simulink model "Master2021b"  (R2021b)
settings: Solver=ode23t  StartTime=0.0  StopTime=simtime  MaxStep=1  RelTol=1e-3
values from neighbouring files (symbols this model uses):
  Af = 1.8    [Akik_DriveCycle_Model_price.m]
  B = 0.0001    [Akik_DriveCycle_Model_price.m]
  Cd = 0.3    [Akik_DriveCycle_Model_price.m]
  Conv_eff = 0.9    [Akik_DriveCycle_Model_price.m]
  fr = 0.015    [Akik_DriveCycle_Model_price.m]
  g = 9.81    [Akik_DriveCycle_Model_price.m]
  Gain = 1    [Akik_DriveCycle_Model_price.m]
  Gr = 9.7    [Akik_DriveCycle_Model_price.m]
  Initial_SOC = 1    [Akik_DriveCycle_Model_price.m]
  J = 1.7    [Akik_DriveCycle_Model_price.m]
  Kd = 0    [Akik_DriveCycle_Model_price.m]
  Ke = 0.33    [Akik_DriveCycle_Model_price.m]
  Ki = 0.05    [Akik_DriveCycle_Model_price.m]
  Kp = 0.3    [Akik_DriveCycle_Model_price.m]
  Kt = 0.33    [Akik_DriveCycle_Model_price.m]
  L = 9e-5    (= 9e-05)    [Akik_DriveCycle_Model_price.m]
  max_brakeT = 3000    [Akik_DriveCycle_Model_price.m]
  Mv = 1500    [Akik_DriveCycle_Model_price.m]
  Qmax = 150    [Akik_DriveCycle_Model_price.m]
  r = 0.35    [Akik_DriveCycle_Model_price.m]
  Ra = 0.55    [Akik_DriveCycle_Model_price.m]
  Rho = 1.2    [Akik_DriveCycle_Model_price.m]
undefined symbols (not defined in the file or in its folder): Ion, Lithium
libraries: simulink x3, spsBatteryLib x1, spsControlledCurrentSourceLib x1, spsStairGeneratorLib x1, spspowerguiLib x1
settings Model: Creator=bkudachi  LastModifiedBy=CP Gaming1
settings DebuggingCC: UnconnectedInputMsg=none  UnconnectedOutputMsg=none  UnconnectedLineMsg=none
settings RTWCC: DLArmComputeVersion=20.02.1

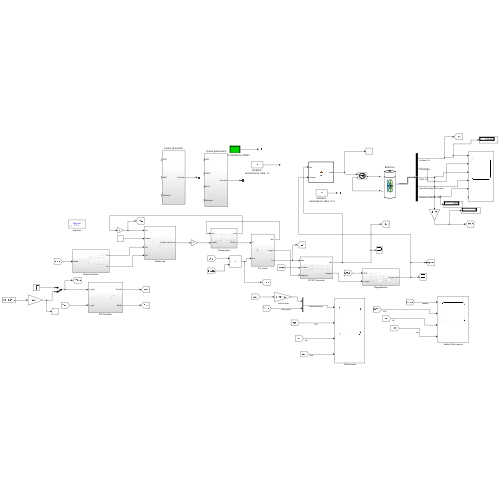
[thumbnail: Simulink's stored preview of the top-level diagram]
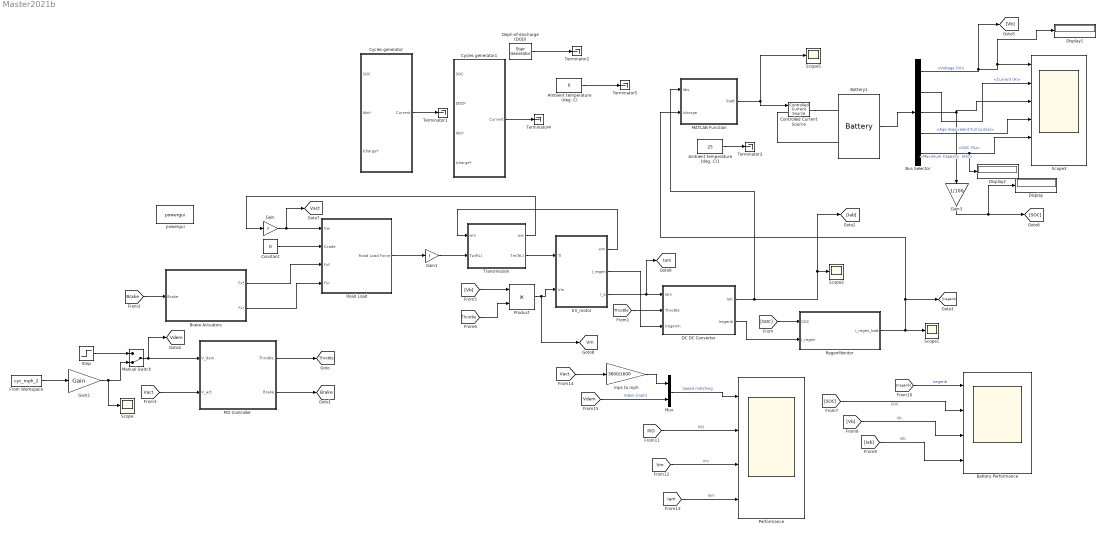
== system Master2021b ==
  " Performance" : Scope  NumInputPorts=4
  Ambient temperature (deg. C) : Constant  Value=0
  Ambient temperature (deg. C)1 : Constant  Value=25
  Battery Performance : Scope  NumInputPorts=4
  Battery1 : spsBatteryLib/Battery  BatType=Lithium-Ion  ShowTempParam=off  ThermalPreset=no  ShowAgeParam=on  NomV=380  NomQ=Qmax  SOC=Initial_SOC*100  Batt_Tr=90  PresetModel=on  MaxQ=150  MinV=285  FullV=442.3151  Dis_rate=65.2174  R=0.025333  Normal_OP=135.6522  expZone="[410.5466      7.369565]"  current=[0.15 1.3 3.25]  Units=Ampere-hour  Tci=25  NomT=20  T2=0  MaxQ2=36  FullV2=13  Normal_OP2=11.7  expZone2="[12.67            4]"  Rca=0.6411  ti=4880  Dp=0  Neq0=0  Tsim=30  Ta1=23  Qeol=40*0.9  Reol=0.0126*1.2  Char_age=[20, 26]  Dis_age=[20, 80]  N1=1500  N2=10445  N3=1017  N4=1460  Ta2=45  N5=982
  Brake Actuators : Subsystem
  Bus Selector : BusSelector  OutputSignals="Voltage (V),Current (A),SOC (%),Age (Equivalent Full cycles),Maximum Capacity  (Ah)"
  Constant : Constant  Value=0
  Controlled Current Source : spsControlledCurrentSourceLib/Controlled Current Source  Initialize=on  Source_Type=AC  Amplitude=0  Phase=0  Frequency=0  Measurements=None
  Cycles generator : Subsystem
  Cycles generator1 : Subsystem
  DC DC Converter : Subsystem
  Deph-of-discharge (DOD) : spsStairGeneratorLib/Stair Generator  t=[0 50 100]*14400  e=[20 80 20]  Ts=0
  Display : Display
  Display1 : Display
  Display2 : Display
  EV_motor : Subsystem
  From Workspace : FromWorkspace  VariableName=cyc_mph_2
  Gain : Gain  Gain=r
  Gain1 : Gain  Gain=r
  Gain2 : Gain  Gain=Gain
  Gain3 : Gain  Gain=1/100
  MATLAB Function : MATLAB Function  TreatAsAtomicUnit=on
  Manual Switch : ManualSwitch  CurrentSetting=0
  Mux : Mux  Inputs=2
  PID Controller : Subsystem
  Product : Product
  RegenMonitor : Subsystem
  Road Load : Subsystem
  Scope{,1..2,5} (4 alike) : Scope
  Scope3 : Scope  NumInputPorts=6
  Step : Step  Time=0  After=100  SampleTime=0
  Terminator{1..5} (5 alike) : Terminator
  Transmission : Subsystem
  mps to mph : Gain  Gain=3600/1600
  powergui : spspowerguiLib/powergui  Priority=1  SimulationMode=Discrete  SampleTime=.1  frequency=60  Iterations=50  frequencyindice=0  Pbase=100e6  ErrMax=1e-4  UnitsV=kV  UnitsW=MW  buscounter=0  FunctionMessages=off  echomessages=off  EnableUseOfTLC=off  CurrentSourceSwitches=off  DisableSnubberDevices=off  DisableRonSwitches=off  DisableVfSwitches=off  DisplayEquations=off  AutomaticDiscreteSolvers=off  SolverType=Tustin/Backward Euler (TBE)  Interpol=off  ExternalGateDelay=off  methode=off  Ts=100  x0status=blocks  SPID=on  SwTol=0  HookPort=off  NonlinearTolerance=1e-4  nMaxIteration=100  ContinueOnMaxIteration=off  RestoreLinks=warning  ResistiveCurrentMeasurement=off  Frange=[0:2:500]  Ylog=off  Xlog=on  ShowGrid=off  save=off  variable=ZData  structure=0  ZoomFFT=off  StartTime=0.0  cycles=1  DisplayStyle=1  fundamental=60  FreqAxis=off  MaxFrequency=1000  frequencyindicesteady=1  RmsSteady=1  display=off
  tag scope: Brake=global, Iam=global, Throttle=global, Vact=global, Vdem=global, Vm=global
  wires:
  Constant/1 -> Road Load/2(Grade)
  Gain/1 -> [Vact], Road Load/1(Vw)
  Road Load/1(Road Load Force) -> Gain1/1
  Brake Actuators/1(Fxf) -> Road Load/3(Fxf)
  Brake Actuators/2(Fxr) -> Road Load/4(Fxr)
  Transmission/1(ww) -> Gain/1
  Transmission/2(Tm(RL)) -> EV_motor/1(Tl)
  EV_motor/1(wm) -> Transmission/1(wm)
  EV_motor/3(I_a) -> [Iam], DC DC Converter/1(Iam)
  EV_motor/2(I_regen) -> DC DC Converter/3(Iregenm)
  DC DC Converter/2(Iregenb) -> RegenMonitor/2(I_regen)
  [SOC] -> RegenMonitor/1(SOC)
  PID Controller/1(Throttle) -> [Throttle]
  PID Controller/2(Brake) -> [Brake]
  RegenMonitor/1(I_regen_batt) -> MATLAB Function/2(Icharge), [Iregenb], Scope1/1
  DC DC Converter/1(Iab) -> MATLAB Function/1(Idis), [Iab], Scope2/1
  [Throttle] -> DC DC Converter/2(Throttle)
  [Brake] -> Brake Actuators/1(Brake)
  [Vact] -> PID Controller/2(V_act)
  [Vb] -> Product/1
  Product/1 -> [Vm], EV_motor/2(Vm)
  [Throttle] -> Product/2
  [Iab] -> Battery Performance/4  "Iab"
  [Iregenb] -> Battery Performance/1  "Iregenb"
  [PID] -> " Performance"/2  "PID"
  [Vm] -> " Performance"/3  "Vm"
  [Iam] -> " Performance"/4  "Iam"
  [Vact] -> mps to mph/1
  mps to mph/1 -> Mux/1
  Mux/1 -> " Performance"/1  "Speed matching"
  [Vdem] -> Mux/2  "Vdem (mph)"
  Step/1 -> Manual Switch/1
  Manual Switch/1 -> [Vdem], PID Controller/1(V_dem)
  From Workspace/1 -> Gain2/1
  Gain2/1 -> Scope/1, Manual Switch/2
  Gain1/1 -> Transmission/2(Tw(RL))
  Battery1/1 -> Bus Selector/1
  Bus Selector/1 -> [Vb], Display1/1, Scope3/1  "<Voltage (V)>"
  Gain3/1 -> Display/1, [SOC]
  [Vb] -> Battery Performance/3  "Vb"
  [SOC] -> Battery Performance/2  "SOC"
  Deph-of-discharge (DOD)/1 -> Terminator2/1
  Cycles generator/1(Current) -> Terminator1/1
  Cycles generator1/1(Current) -> Terminator4/1
  Ambient temperature (deg. C)/1 -> Terminator5/1
  MATLAB Function/1(ibatt) -> Scope5/1, Controlled Current Source/1
  Bus Selector/2 -> Scope3/2  "<Current (A)>"
  Bus Selector/3 -> Scope3/3, Gain3/1  "<SOC (%)>"
  Ambient temperature (deg. C)1/1 -> Terminator3/1
  Bus Selector/4 -> Scope3/4  "<Age (Equivalent Full cycles)>"
  Bus Selector/5 -> Display2/1, Scope3/5  "<Maximum Capacity  (Ah)>"
  connections:
  Controlled Current Source/RConn1 -- Battery1/LConn2
  Controlled Current Source/LConn1 -- Battery1/LConn1

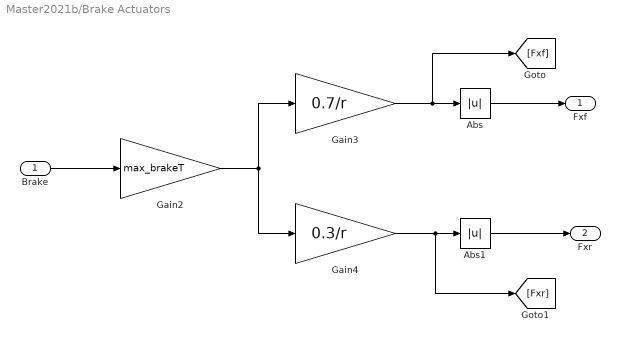
== system Master2021b/Brake Actuators ==
  Brake : Inport
  Abs : Abs
  Abs1 : Abs
  Gain2 : Gain  Gain=max_brakeT
  Gain3 : Gain  Gain=0.7/r
  Gain4 : Gain  Gain=0.3/r
  Fxf : Outport
  Fxr : Outport  Port=2
  wires:
  Gain3/1 -> Abs/1, [Fxf]
  Gain4/1 -> [Fxr], Abs1/1
  Abs1/1 -> Fxr/1
  Gain2/1 -> Gain3/1, Gain4/1
  Brake/1 -> Gain2/1
  Abs/1 -> Fxf/1

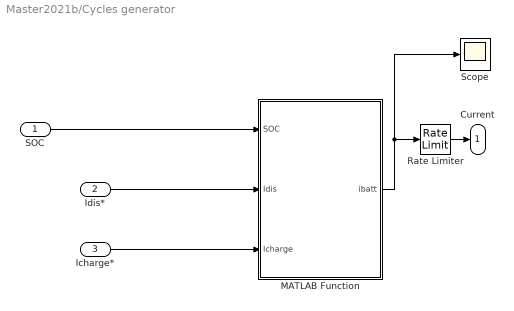
== system Master2021b/Cycles generator ==
  SOC : Inport
  Idis* : Inport  Port=2
  Icharge* : Inport  Port=3
  MATLAB Function : MATLAB Function  TreatAsAtomicUnit=on
  Rate Limiter : RateLimiter  RisingSlewLimit=1000  FallingSlewLimit=-1000  SampleTimeMode=inherited
  Scope : Scope
  Current : Outport  VectorParamsAs1DForOutWhenUnconnected=off
  wires:
  MATLAB Function/1(ibatt) -> Scope/1, Rate Limiter/1
  Idis*/1 -> MATLAB Function/2(Idis)
  Icharge*/1 -> MATLAB Function/3(Icharge)
  Rate Limiter/1 -> Current/1
  SOC/1 -> MATLAB Function/1(SOC)

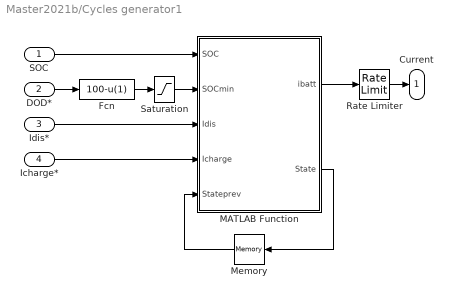
== system Master2021b/Cycles generator1 ==
  SOC : Inport
  DOD* : Inport  Port=2
  Idis* : Inport  Port=3
  Icharge* : Inport  Port=4
  Fcn : Fcn  Expr=100-u(1)
  MATLAB Function : MATLAB Function  TreatAsAtomicUnit=on
  Memory : Memory  InitialCondition=1
  Rate Limiter : RateLimiter  RisingSlewLimit=1000  FallingSlewLimit=-1000  SampleTimeMode=inherited
  Saturation : Saturate  UpperLimit=98  LowerLimit=1
  Current : Outport  VectorParamsAs1DForOutWhenUnconnected=off
  wires:
  MATLAB Function/1(ibatt) -> Rate Limiter/1
  SOC/1 -> MATLAB Function/1(SOC)
  Memory/1 -> MATLAB Function/5(Stateprev)
  MATLAB Function/2(State) -> Memory/1
  DOD*/1 -> Fcn/1
  Fcn/1 -> Saturation/1
  Saturation/1 -> MATLAB Function/2(SOCmin)
  Idis*/1 -> MATLAB Function/3(Idis)
  Icharge*/1 -> MATLAB Function/4(Icharge)
  Rate Limiter/1 -> Current/1

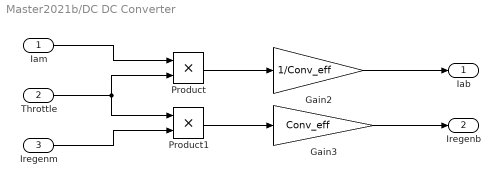
== system Master2021b/DC DC Converter ==
  Iam : Inport
  Throttle : Inport  Port=2
  Iregenm : Inport  Port=3
  Gain2 : Gain  Gain=1/Conv_eff
  Gain3 : Gain  Gain=Conv_eff
  Product : Product
  Product1 : Product
  Iab : Outport
  Iregenb : Outport  Port=2
  wires:
  Throttle/1 -> Product1/1, Product/2
  Gain3/1 -> Iregenb/1
  Gain2/1 -> Iab/1
  Product1/1 -> Gain3/1
  Iam/1 -> Product/1
  Iregenm/1 -> Product1/2
  Product/1 -> Gain2/1

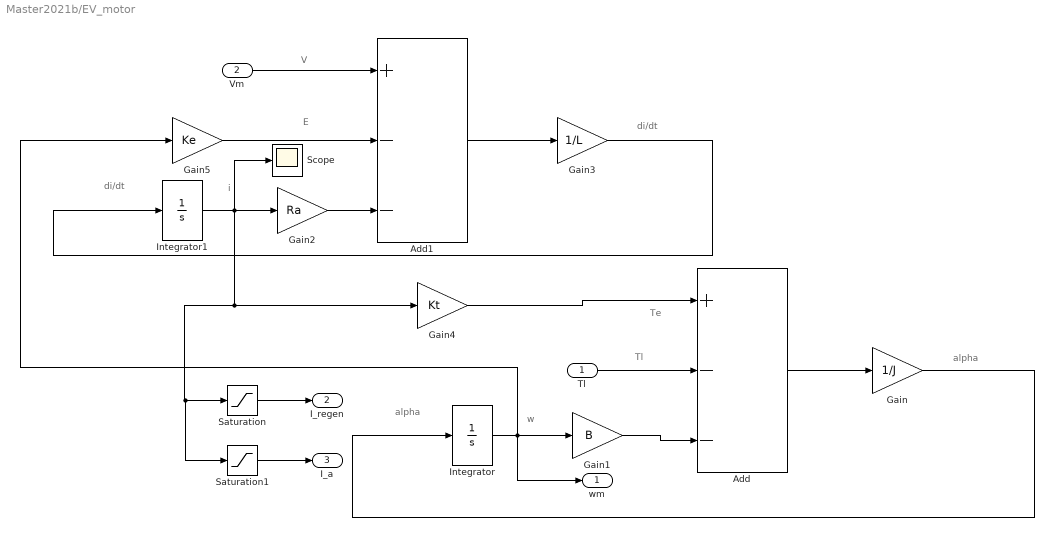
== system Master2021b/EV_motor ==
  note: di/dt
  note: E
  note: V
  note: i
  note: di/dt
  note: alpha
  note: Tl
  note: Te
  note: w
  note: alpha
  Tl : Inport
  Vm : Inport  Port=2
  Add : Sum  Inputs=+--
  Add1 : Sum  Inputs=+--
  Gain : Gain  Gain=1/J
  Gain1 : Gain  Gain=B
  Gain2 : Gain  Gain=Ra
  Gain3 : Gain  Gain=1/L
  Gain4 : Gain  Gain=Kt
  Gain5 : Gain  Gain=Ke
  Integrator : Integrator
  Integrator1 : Integrator
  Saturation : Saturate  UpperLimit=0  LowerLimit=-inf
  Saturation1 : Saturate  UpperLimit=inf  LowerLimit=0
  Scope : Scope
  wm : Outport
  I_regen : Outport  Port=2
  I_a : Outport  Port=3
  wires:
  Integrator/1 -> wm/1, Gain5/1, Gain1/1
  Add/1 -> Gain/1
  Gain1/1 -> Add/3
  Gain/1 -> Integrator/1
  Gain3/1 -> Integrator1/1
  Integrator1/1 -> Scope/1, Saturation1/1, Saturation/1, Gain4/1, Gain2/1
  Vm/1 -> Add1/1
  Gain2/1 -> Add1/3
  Add1/1 -> Gain3/1
  Gain4/1 -> Add/1
  Gain5/1 -> Add1/2
  Tl/1 -> Add/2
  Saturation/1 -> I_regen/1
  Saturation1/1 -> I_a/1

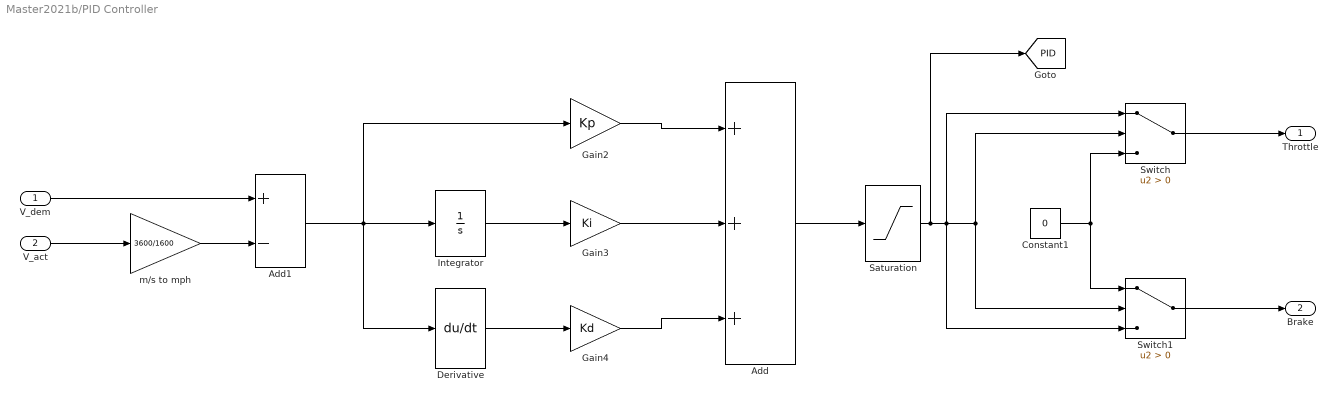
== system Master2021b/PID Controller ==
  V_dem : Inport
  V_act : Inport  Port=2
  Add : Sum  Inputs=+++
  Add1 : Sum  Inputs=+-
  Constant1 : Constant  Value=0
  Derivative : Derivative
  Gain2 : Gain  Gain=Kp
  Gain3 : Gain  Gain=Ki
  Gain4 : Gain  Gain=Kd
  Integrator : Integrator
  Saturation : Saturate  UpperLimit=1  LowerLimit=-1
  Switch : Switch  Criteria=u2 > Threshold
  Switch1 : Switch  Criteria=u2 > Threshold
  m/s to mph : Gain  Gain=3600/1600
  Throttle : Outport
  Brake : Outport  Port=2
  tag scope: PID=global
  wires:
  V_act/1 -> m/s to mph/1
  Saturation/1 -> [PID], Switch1/3, Switch/1, Switch1/2, Switch/2
  Integrator/1 -> Gain3/1
  Constant1/1 -> Switch/3, Switch1/1
  Switch/1 -> Throttle/1
  V_dem/1 -> Add1/1
  Derivative/1 -> Gain4/1
  Switch1/1 -> Brake/1
  Gain3/1 -> Add/2
  m/s to mph/1 -> Add1/2
  Add/1 -> Saturation/1
  Gain2/1 -> Add/1
  Gain4/1 -> Add/3
  Add1/1 -> Derivative/1, Gain2/1, Integrator/1

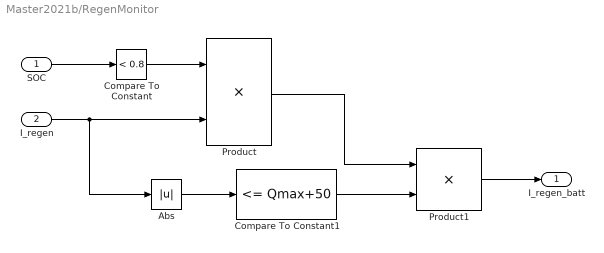
== system Master2021b/RegenMonitor ==
  SOC : Inport
  I_regen : Inport  Port=2
  Abs : Abs
  Compare To Constant : simulink/Logic and Bit Operations/Compare To Constant  relop=<  const=0.8  OutDataTypeStr=boolean
  Compare To Constant1 : simulink/Logic and Bit Operations/Compare To Constant  relop=<=  const=Qmax+50  OutDataTypeStr=boolean
  Product : Product
  Product1 : Product
  I_regen_batt : Outport
  wires:
  Product1/1 -> I_regen_batt/1
  Product/1 -> Product1/1
  SOC/1 -> Compare To Constant/1
  I_regen/1 -> Abs/1, Product/2
  Abs/1 -> Compare To Constant1/1
  Compare To Constant/1 -> Product/1
  Compare To Constant1/1 -> Product1/2

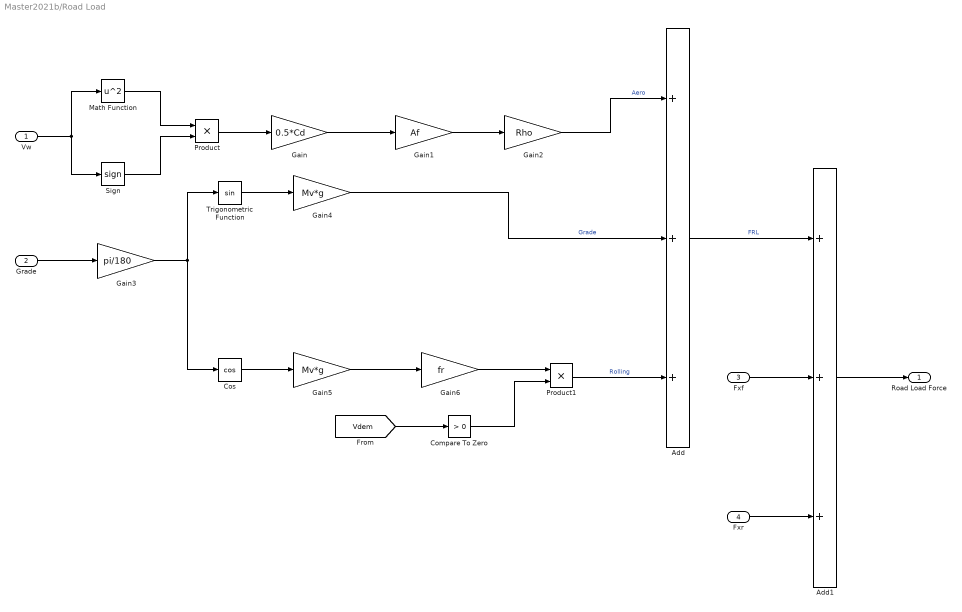
== system Master2021b/Road Load ==
  Vw : Inport
  Grade : Inport  Port=2
  Fxf : Inport  Port=3
  Fxr : Inport  Port=4
  Add : Sum  Inputs=+++
  Add1 : Sum  Inputs=+++
  Compare To Zero : simulink/Logic and Bit Operations/Compare To Zero  relop=>  OutDataTypeStr=boolean
  Cos : Trigonometry  Operator=cos
  Gain : Gain  Gain=0.5*Cd
  Gain1 : Gain  Gain=Af
  Gain2 : Gain  Gain=Rho
  Gain3 : Gain  Gain=pi/180
  Gain4 : Gain  Gain=Mv*g
  Gain5 : Gain  Gain=Mv*g
  Gain6 : Gain  Gain=fr
  Math Function : Math  Operator=square  SaturateOnIntegerOverflow=on
  Product : Product
  Product1 : Product
  Sign : Signum
  Trigonometric Function : Trigonometry
  Road Load Force : Outport
  wires:
  Gain/1 -> Gain1/1
  Grade/1 -> Gain3/1
  Gain4/1 -> Add/2  "Grade"
  Math Function/1 -> Product/1
  Product/1 -> Gain/1
  Vw/1 -> Math Function/1, Sign/1
  Gain2/1 -> Add/1  "Aero"
  Gain3/1 -> Trigonometric Function/1, Cos/1
  Gain1/1 -> Gain2/1
  Gain6/1 -> Product1/1
  Cos/1 -> Gain5/1
  Sign/1 -> Product/2
  Trigonometric Function/1 -> Gain4/1
  Gain5/1 -> Gain6/1
  Product1/1 -> Add/3  "Rolling"
  Add/1 -> Add1/1  "FRL"
  Compare To Zero/1 -> Product1/2
  [Vdem] -> Compare To Zero/1
  Fxf/1 -> Add1/2
  Fxr/1 -> Add1/3
  Add1/1 -> Road Load Force/1

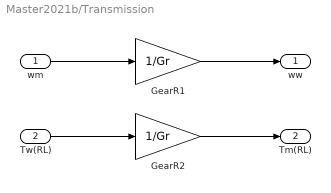
== system Master2021b/Transmission ==
  wm : Inport
  Tw(RL) : Inport  Port=2
  GearR1 : Gain  Gain=1/Gr
  GearR2 : Gain  Gain=1/Gr
  ww : Outport
  Tm(RL) : Outport  Port=2
  wires:
  GearR1/1 -> ww/1
  Tw(RL)/1 -> GearR2/1
  wm/1 -> GearR1/1
  GearR2/1 -> Tm(RL)/1

== matlab function Master2021b/Cycles generator1/MATLAB Function ==
  data: SOC input; SOCmin input; Idis input; Icharge input; ibatt output; Stateprev input; State output
function [ibatt,State] = fcn(SOC,SOCmin,Idis,Icharge,Stateprev)
%#codegen
State=Stateprev;
if(Stateprev==1 && SOC<=SOCmin)
    State=0;
end
if(Stateprev==0 && SOC>=99)
    State=1;
end
if (Stateprev==1)
    ibatt=Idis;
else
    ibatt=-Icharge;
end

== matlab function Master2021b/Cycles generator/MATLAB Function ==
  data: SOC input; Idis input; Icharge input; ibatt output
function ibatt = fcn(SOC,Idis,Icharge)
%#codegen
%State=Stateprev;
% if(Stateprev==1 && SOC<=SOCmin)
%     State=0;
% end
% if(Stateprev==0 && SOC>=99)
%      State=1;
% end
if (SOC>=0.2 && SOC<=0.8)
    ibatt=Idis;
else
    ibatt=-Icharge;
end

== matlab function Master2021b/MATLAB Function ==
  data: Idis input; ibatt output; Icharge input
function ibatt  = fcn(Idis,Icharge)

if Idis>0
    ibatt = Idis;
else
    ibatt = -Icharge;
end
